simulink model "Lab4SimulinkStep"  (R2018b)
settings: Solver=VariableStepAuto  StartTime=0.0  StopTime=5  RelTol=1e-6
libraries: simulink x2
settings Model: Creator=rahul  LastModifiedBy=Keyanna
settings DebuggingCC: LibraryContextMissingDiagnostic=none
settings SFSimCC: SimUseLocalCustomCode=off
settings RTWCC: RTWUseLocalCustomCode=off

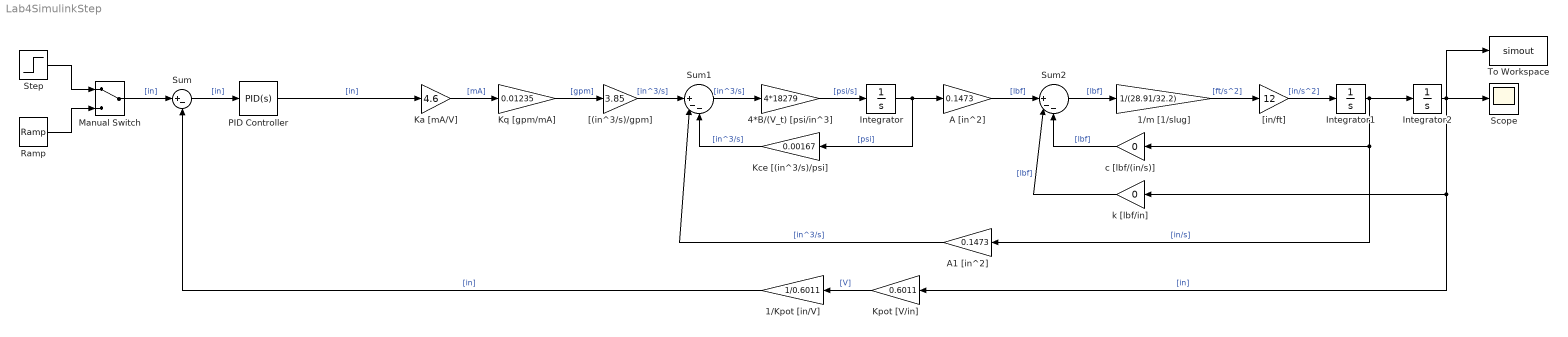
== system Lab4SimulinkStep ==
  1/Kpot [in/V] : Gain  Gain=1/0.6011
  1/m [1/slug] : Gain  Gain=1/(28.91/32.2)
  4*B/(V_t) [psi/in^3] : Gain  Gain=4*18279
  A [in^2] : Gain  Gain=0.1473
  A1 [in^2] : Gain  Gain=0.1473
  Integrator : Integrator
  Integrator1 : Integrator
  Integrator2 : Integrator
  Ka [mA/V] : Gain  Gain=4.6
  Kce [(in^3/s)/psi] : Gain  Gain=0.00167
  Kpot [V/in] : Gain  Gain=0.6011
  Kq [gpm/mA] : Gain  Gain=0.01235
  Manual Switch : ManualSwitch
  PID Controller : simulink/Continuous/PID Controller  Controller=PID  Form=Parallel  TimeDomain=Continuous-time  SampleTime=-1  IntegratorMethod=Forward Euler  FilterMethod=Forward Euler  ControllerParametersSource=internal  P=82  I=0  D=0  UseFilter=on  N=100  TunerSelectOption=Transfer Function Based (PID Tuner App)  InitialConditionSource=internal  InitialConditionForIntegrator=0  InitialConditionForFilter=0  DifferentiatorICPrevScaledInput=0  ExternalReset=none  TrackingMode=off  Kt=1  LimitOutput=off  UpperSaturationLimit=inf  LowerSaturationLimit=-inf  LinearizeAsGain=on  AntiWindupMode=none  Kb=1  POutMin=[]  POutMax=[]  IOutMin=[]  IOutMax=[]  DOutMin=[]  DOutMax=[]  NOutMin=[]  NOutMax=[]  SumOutMin=[]  SumOutMax=[]  SaturationOutMin=[]  SaturationOutMax=[]  PParamMin=[]  PParamMax=[]  IParamMin=[]  IParamMax=[]  DParamMin=[]  DParamMax=[]  NParamMin=[]  NParamMax=[]  KbParamMin=[]  KbParamMax=[]  KtParamMin=[]  KtParamMax=[]  KbOutMin=[]  KbOutMax=[]  KtOutMin=[]  KtOutMax=[]  IntegratorOutMin=[]  IntegratorOutMax=[]  FilterOutMin=[]  FilterOutMax=[]  SumI1OutMin=[]  SumI1OutMax=[]  SumI2OutMin=[]  SumI2OutMax=[]  SumI3OutMin=[]  SumI3OutMax=[]  SumI4OutMin=[]  SumI4OutMax=[]  SumDOutMin=[]  SumDOutMax=[]  DifferentiatorOutMin=[]  DifferentiatorOutMax=[]  FilterDiffOutCoefMin=[]  FilterDiffOutCoefMax=[]  ReciprocalOutMin=[]  ReciprocalOutMax=[]  SumDenOutMin=[]  SumDenOutMax=[]  SumNumOutMin=[]  SumNumOutMax=[]  DivideOutMin=[]  DivideOutMax=[]  IntegratorContinuousStateAttributes=''  IntegratorStateMustResolveToSignalObject=off  IntegratorRTWStateStorageClass=Auto  FilterContinuousStateAttributes=''  FilterStateMustResolveToSignalObject=off  FilterRTWStateStorageClass=Auto  ParallelPVariant=InternalParameters  IdealPVariant=Disabled  IVariant=InternalParameters  DVariant=InternalParameters  IntegratorVariant=Continuous  SatVariant=Disabled  AWVariant=Passthrough  PCopyVariant=Disabled  TRVariant=Disabled  FdbkBlocksVariant=Forward  IdealPFdbkVariant=Disabled  SatFdbkVariant=Disabled  DerivativeFilterVariant=ContFilter  NVariant=InternalParameters  NCopyVariant=Disabled  FilterICVariant=InternalICsFilter  IntegratorICVariant=InternalICs  ExternalResetVariant=Disabled  TRSumVariant=Passthrough  SumFdbkVariant=Disabled  SumVariant=Sum_PID
  Ramp : simulink/Sources/Ramp  slope=1  start=0  InitialOutput=0
  Scope : Scope
  Step : Step  SampleTime=0
  Sum : Sum  Inputs=|+-
  Sum1 : Sum  Inputs=||+--
  Sum2 : Sum  Inputs=||+--
  To Workspace : ToWorkspace  VariableName=simout  SampleTime=-1
  "[(in^3/s)/gpm]" : Gain  Gain=3.85
  "[in/ft]" : Gain  Gain=12
  c [lbf/(in/s)] : Gain  Gain=0
  k [lbf/in] : Gain  Gain=0
  wires:
  Manual Switch/1 -> Sum/1  "[in]"
  Ka [mA/V]/1 -> Kq [gpm/mA]/1  "[mA]"
  Sum1/1 -> 4*B/(V_t) [psi/in^3]/1  "[in^3/s]"
  4*B/(V_t) [psi/in^3]/1 -> Integrator/1  "[psi/s]"
  Integrator/1 -> Kce [(in^3/s)/psi]/1, A [in^2]/1  "[psi]"
  A [in^2]/1 -> Sum2/1  "[lbf]"
  Sum2/1 -> 1/m [1/slug]/1  "[lbf]"
  Integrator1/1 -> A1 [in^2]/1, c [lbf/(in/s)]/1, Integrator2/1  "[in/s]"
  Integrator2/1 -> To Workspace/1, Kpot [V/in]/1, k [lbf/in]/1, Scope/1  "[in]"
  c [lbf/(in/s)]/1 -> Sum2/3  "[lbf]"
  k [lbf/in]/1 -> Sum2/2  "[lbf]"
  A1 [in^2]/1 -> Sum1/2  "[in^3/s]"
  Kce [(in^3/s)/psi]/1 -> Sum1/3  "[in^3/s]"
  Kpot [V/in]/1 -> 1/Kpot [in/V]/1  "[V]"
  1/Kpot [in/V]/1 -> Sum/2  "[in]"
  PID Controller/1 -> Ka [mA/V]/1  "[in]"
  Sum/1 -> PID Controller/1  "[in]"
  "[(in^3/s)/gpm]"/1 -> Sum1/1  "[in^3/s]"
  Kq [gpm/mA]/1 -> "[(in^3/s)/gpm]"/1  "[gpm]"
  1/m [1/slug]/1 -> "[in/ft]"/1  "[ft/s^2]"
  "[in/ft]"/1 -> Integrator1/1  "[in/s^2]"
  Step/1 -> Manual Switch/1
  Ramp/1 -> Manual Switch/2
